simulink model "item2ModeloNLin"  (R2017a)
settings: Solver=VariableStepAuto  StartTime=0.0  StopTime=50  RelTol=1e-3
libraries: simulink x6
settings Model: Creator=julia  LastModifiedBy=julia

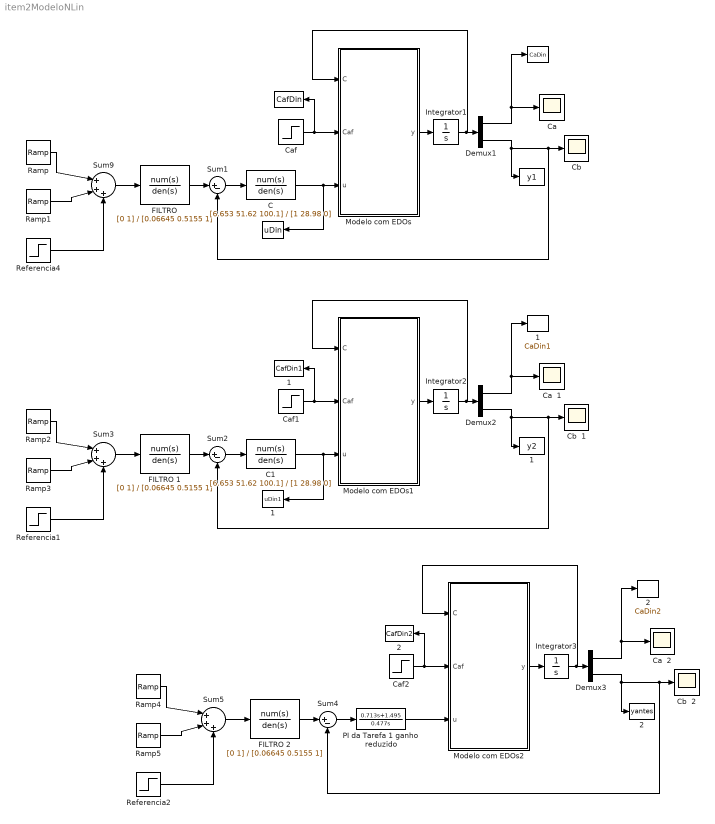
== system item2ModeloNLin ==
  "   " : ToWorkspace  VariableName=y1  SaveFormat=Timeseries  SampleTime=-1
  "          " : ToWorkspace  VariableName=CafDin  SaveFormat=Timeseries  SampleTime=-1
  "                 " : ToWorkspace  VariableName=uDin  SaveFormat=Timeseries  SampleTime=-1
  "                   " : ToWorkspace  VariableName=CaDin  SaveFormat=Timeseries  SampleTime=-1
  "                   1" : ToWorkspace  VariableName=CaDin1  SaveFormat=Timeseries  SampleTime=-1
  "                   2" : ToWorkspace  VariableName=CaDin2  SaveFormat=Timeseries  SampleTime=-1
  "                 1" : ToWorkspace  VariableName=uDin1  SaveFormat=Timeseries  SampleTime=-1
  "          1" : ToWorkspace  VariableName=CafDin1  SaveFormat=Timeseries  SampleTime=-1
  "          2" : ToWorkspace  VariableName=CafDin2  SaveFormat=Timeseries  SampleTime=-1
  "   1" : ToWorkspace  VariableName=y2  SaveFormat=Timeseries  SampleTime=-1
  "   2" : ToWorkspace  VariableName=yantes  SaveFormat=Timeseries  SampleTime=-1
  C : TransferFcn  Numerator=[6.653 51.62 100.1]  Denominator=[1 28.98 0]
  C1 : TransferFcn  Numerator=[6.653 51.62 100.1]  Denominator=[1 28.98 0]
  "Ca  " : Scope
  Ca  1 : Scope
  Ca  2 : Scope
  Caf : Step  Time=35  Before=5.1  After=5.15  SampleTime=0
  Caf1 : Step  Time=35  Before=5.1  After=5.15  SampleTime=0
  Caf2 : Step  Time=35  Before=5.1  After=5.15  SampleTime=0
  "Cb  " : Scope
  Cb  1 : Scope
  Cb  2 : Scope
  Demux1 : Demux  Outputs=2
  Demux2 : Demux  Outputs=2
  Demux3 : Demux  Outputs=2
  "FILTRO " : TransferFcn  Numerator=[0 1]  Denominator=[0.06645 0.5155 1]
  FILTRO 1 : TransferFcn  Numerator=[0 1]  Denominator=[0.06645 0.5155 1]
  FILTRO 2 : TransferFcn  Numerator=[0 1]  Denominator=[0.06645 0.5155 1]
  Integrator1 : Integrator  InitialCondition=[0;0]
  Integrator2 : Integrator  InitialCondition=[0;0]
  Integrator3 : Integrator  InitialCondition=[0;0]
  Modelo com EDOs : MATLAB Function  TreatAsAtomicUnit=on
  Modelo com EDOs1 : MATLAB Function  TreatAsAtomicUnit=on
  Modelo com EDOs2 : MATLAB Function  TreatAsAtomicUnit=on
  PI da Tarefa 1 ganho reduzido : TransferFcn  Numerator="[0.713  1.495]"  Denominator=[0.477 0]
  Ramp : simulink/Sources/Ramp  slope=2.345/10  start=0  X0=0
  Ramp1 : simulink/Sources/Ramp  slope=-2.345/10  start=10  X0=0
  Ramp2 : simulink/Sources/Ramp  slope=2.345/10  start=0  X0=0
  Ramp3 : simulink/Sources/Ramp  slope=-2.345/10  start=10  X0=0
  Ramp4 : simulink/Sources/Ramp  slope=2.345/10  start=0  X0=0
  Ramp5 : simulink/Sources/Ramp  slope=-2.345/10  start=10  X0=0
  Referencia1 : Step  Time=20  After=0.35  SampleTime=0
  Referencia2 : Step  Time=20  After=0.35  SampleTime=0
  Referencia4 : Step  Time=20  After=0.25  SampleTime=0
  Sum1 : Sum  Inputs=|+-
  Sum2 : Sum  Inputs=|+-
  Sum3 : Sum  Inputs=|+++
  Sum4 : Sum  Inputs=|+-
  Sum5 : Sum  Inputs=|+++
  Sum9 : Sum  Inputs=|+++
  wires:
  Modelo com EDOs/1(y) -> Integrator1/1
  Integrator1/1 -> Modelo com EDOs/1(C), Demux1/1
  C/1 -> "                 "/1, Modelo com EDOs/3(u)
  Demux1/1 -> "                   "/1, "Ca  "/1
  "FILTRO "/1 -> Sum1/1
  Sum1/1 -> C/1
  Demux1/2 -> "Cb  "/1, Sum1/2, "   "/1
  Caf/1 -> "          "/1, Modelo com EDOs/2(Caf)
  Referencia4/1 -> Sum9/3
  Sum9/1 -> "FILTRO "/1
  Ramp1/1 -> Sum9/2
  Ramp/1 -> Sum9/1
  Ramp2/1 -> Sum3/1
  Ramp3/1 -> Sum3/2
  Sum3/1 -> FILTRO 1/1
  Referencia1/1 -> Sum3/3
  Caf1/1 -> Modelo com EDOs1/2(Caf), "          1"/1
  Demux2/2 -> "   1"/1, Sum2/2, Cb  1/1
  Sum2/1 -> C1/1
  FILTRO 1/1 -> Sum2/1
  Demux2/1 -> Ca  1/1, "                   1"/1
  C1/1 -> Modelo com EDOs1/3(u), "                 1"/1
  Integrator2/1 -> Demux2/1, Modelo com EDOs1/1(C)
  Modelo com EDOs1/1(y) -> Integrator2/1
  Modelo com EDOs2/1(y) -> Integrator3/1
  Integrator3/1 -> Modelo com EDOs2/1(C), Demux3/1
  PI da Tarefa 1 ganho reduzido/1 -> Modelo com EDOs2/3(u)
  Demux3/1 -> "                   2"/1, Ca  2/1
  FILTRO 2/1 -> Sum4/1
  Sum4/1 -> PI da Tarefa 1 ganho reduzido/1
  Demux3/2 -> Cb  2/1, Sum4/2, "   2"/1
  Caf2/1 -> "          2"/1, Modelo com EDOs2/2(Caf)
  Referencia2/1 -> Sum5/3
  Sum5/1 -> FILTRO 2/1
  Ramp5/1 -> Sum5/2
  Ramp4/1 -> Sum5/1

== matlab function item2ModeloNLin/Modelo com EDOs ==
  data: y output; C input; Caf input; u input
%EDOs das concentracoes dos produtos A e B
function y = fcn(C, Caf, u)

%constantes
k1 = 6.01; %L/min
k2 = 0.8433; %L/min
k3 = 0.1123; %mol/Lmin

%variaveis das concentracoes dos produtos A e B
Ca = C(1);
Cb = C(2);

%EDOs
Ca_d = -k1*Ca - k3*(Ca^2) + (Caf - Ca)*u;
Cb_d =  k1*Ca - k2*Cb - Cb*u;
 
%conjunto das EDOs
y = [Ca_d;Cb_d];

== matlab function item2ModeloNLin/Modelo com EDOs1 ==
  data: y output; C input; Caf input; u input
%EDOs das concentracoes dos produtos A e B
function y = fcn(C, Caf, u)

%constantes
k1 = 6.01; %L/min
k2 = 0.8433; %L/min
k3 = 0.1123; %mol/Lmin

%variaveis das concentracoes dos produtos A e B
Ca = C(1);
Cb = C(2);

%EDOs
Ca_d = -k1*Ca - k3*(Ca^2) + (Caf - Ca)*u;
Cb_d =  k1*Ca - k2*Cb - Cb*u;
 
%conjunto das EDOs
y = [Ca_d;Cb_d];

== matlab function item2ModeloNLin/Modelo com EDOs2 ==
  data: y output; C input; Caf input; u input
%EDOs das concentracoes dos produtos A e B
function y = fcn(C, Caf, u)

%constantes
k1 = 6.01; %L/min
k2 = 0.8433; %L/min
k3 = 0.1123; %mol/Lmin

%variaveis das concentracoes dos produtos A e B
Ca = C(1);
Cb = C(2);

%EDOs
Ca_d = -k1*Ca - k3*(Ca^2) + (Caf - Ca)*u;
Cb_d =  k1*Ca - k2*Cb - Cb*u;
 
%conjunto das EDOs
y = [Ca_d;Cb_d];
